simulink model "Loops4"  (Simulink 6.0)
settings: Solver=ode45  StartTime=0.0  StopTime=10.0  RelTol=1e-3
settings Model: Creator=scaife  LastModifiedBy=scaife  ExtModeAutoUpdateStatusClock=off
settings DataIOCC: SignalLoggingName=sigsOut
settings DebuggingCC: SolverPrmCheckMsg=none
settings HardwareCC: TargetUnknown=on
settings GRTTargetCC: ModelReferenceCompliant=off  MatFileLogging=off

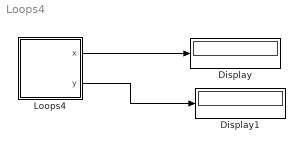
== system Loops4 ==
  Display : Display
  Display1 : Display
  Loops4 : Stateflow chart
  wires:
  Loops4/1(x) -> Display/1
  Loops4/2(y) -> Display1/1

== stateflow chart Loops4 ==
  state A
  state B
  A -> (junction 5) : {x=0;}
  (junction 6) -> B
  (default) -> A
  (junction 7) -> B
  (junction 5) -> (junction 6) : [!y]
  (junction 5) -> (junction 7) : [y]
  (junction 7) -> (junction 7) : [x<5]
      | {x++;}
  (junction 6) -> (junction 6) : [x<10]
      | {x++;}
  B -> A : {y=!y}
  data: x output int32; y output boolean
